simulink model "reactor"  (R2021a)
settings: Solver=VariableStepAuto  StartTime=0.0  StopTime=10.0  RelTol=1e-3
settings Model: Creator=Automatica  LastModifiedBy=Automatica

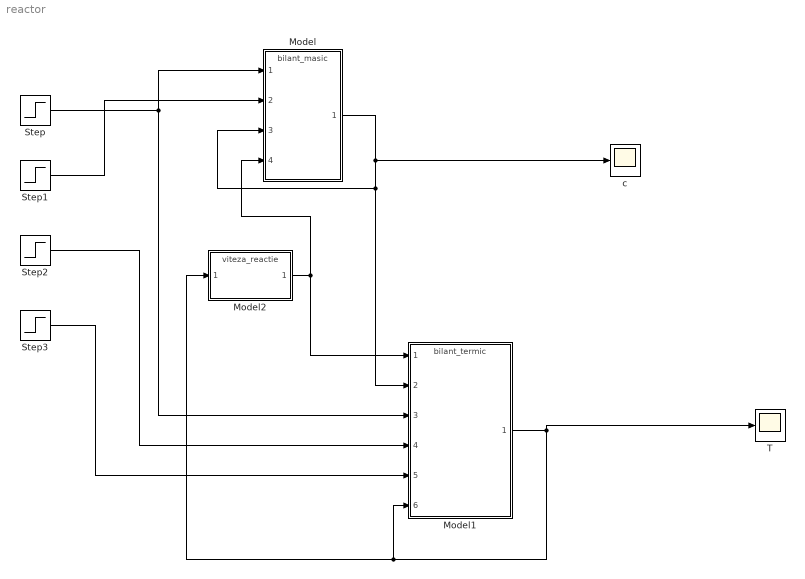
== system reactor ==
  Model : ModelReference  ModelNameDialog=bilant_masic.slx  SimulationMode=Normal  ModelReferenceVersion=1.5
  Model1 : ModelReference  ModelNameDialog=bilant_termic.slx  SimulationMode=Normal  ModelReferenceVersion=1.4
  Model2 : ModelReference  ModelNameDialog=viteza_reactie.slx  SimulationMode=Normal  ModelReferenceVersion=1.6
  Step{,1..3} (4 alike) : Step  SampleTime=0
  T : Scope
  c : Scope
  wires:
  Step/1 -> Model1/3, Model/1
  Step1/1 -> Model/2
  Step2/1 -> Model1/4
  Model2/1 -> Model/4, Model1/1
  Model/1 -> c/1, Model1/2, Model/3
  Model1/1 -> T/1, Model2/1, Model1/6
  Step3/1 -> Model1/5
